simulink model "quad_sim_outerloop_multiple_UAVs_pyramid"  (R2017a)
settings: Solver=VariableStepAuto  StartTime=0.0  StopTime=250  FixedStep=0.025  MaxStep=0.03  MinStep=0.02  RelTol=1e-3  EnableMultiTasking=on
InitFcn:
  | setup_gains
  | % --- Outer loop gains --------
  | %P_X=9.44;   I_X=0.23;  D_X=2.36;
  | %P_Y=9.33;   I_Y=0.18;  D_Y=1.54;
  | % --------------------------
  | 
  | %CARLA TUNNED PID
  | %P_Z = 51.037;       I_Z = 43.051;        D_Z = 11.771;
  | %P_Z = 0.5;       I_Z = 0.15;        D_Z = 0.2;
  | %P_Z = 32.55;       I_Z = 9.82;        D_Z = 4.65 ;
  | 
  | global clientID;
  | clientID=-1;
values from neighbouring files (symbols this model uses):
  End_POS_pyramid = [ 0.3000 1.3000 0.000 ... (first row only)    [setup_gains.m]
  Kd_az = 0.001    [setup_gains.m]
  Kd_px = 0.5    [setup_gains.m]
  Kd_py = 0.5    [setup_gains.m]
  Kd_pz = 0.025    [setup_gains.m]
  Kd_vx = 2    [setup_gains.m]
  Kd_vy = 2    [setup_gains.m]
  Kd_vz = 0.05    [setup_gains.m]
  Ki_az = 0.01    [setup_gains.m]
  Ki_px = 0.001    [setup_gains.m]
  Ki_py = 0.001    [setup_gains.m]
  Ki_pz = 0.001    [setup_gains.m]
  Ki_vx = 0.1    [setup_gains.m]
  Ki_vy = 0.1    [setup_gains.m]
  Ki_vz = 2.5    [setup_gains.m]
  Kp_az = 0.75    [setup_gains.m]
  Kp_px = 1    [setup_gains.m]
  Kp_py = 1    [setup_gains.m]
  Kp_pz = 0.5    [setup_gains.m]
  Kp_vx = 15.00    (= 15)    [setup_gains.m]
  Kp_vy = 15.00    (= 15)    [setup_gains.m]
  Kp_vz = 5    [setup_gains.m]
  Start_POS = [ 0.0 0.00 1.00 ... (first row only)    [setup_gains.m]
undefined symbols (not defined in the file or in its folder): W, X, Y, Z
libraries: robotlib x27, dspindex x27, dspsigops x27, simulink x27
(part 1 of 3)
settings Model: Creator=Kleber Cabral  LastModifiedBy=Kleber Cabral
settings DataIOCC: SaveFormat=Array
settings OptimizationCC: LifeSpan=inf
settings DebuggingCC: SolverPrmCheckMsg=warning  SFUnexpectedBacktrackingDiag=warning  SFNoUnconditionalDefaultTransitionDiag=warning  SFExecutionAtInitializationDiag=none
settings HardwareCC: ProdBitPerPointer=32  ProdBitPerSizeT=32  ProdBitPerPtrDiffT=32  ProdLargestAtomicFloat=None  ProdIntDivRoundTo=Undefined  ProdEndianess=Unspecified  ProdWordSize=32  ProdHWDeviceType=32-bit Generic
settings ModelReferenceCC: PropagateSignalLabelsOutOfModel=off
settings GRTTargetCC: TargetLangStandard=C89/C90 (ANSI)  GeneratePreprocessorConditionals=Disable all
settings ConfigComp: CovMetricSettings=dw  CovHtmlReporting=on  CovSaveCumulativeToWorkspaceVar=on  CovSaveSingleToWorkspaceVar=on  CovExternalEMLEnable=off  CovSFcnEnable=off

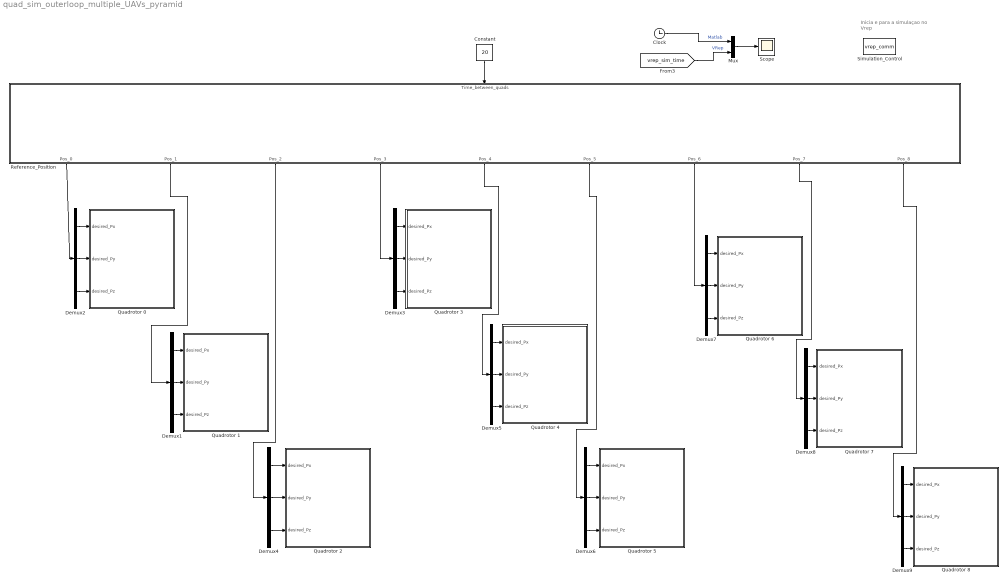
== system quad_sim_outerloop_multiple_UAVs_pyramid ==
  note: Inicia e para a simulaçao no Vrep
  Clock : Clock
  Constant : Constant  Value=20
  Demux{1..9} (9 alike) : Demux  Outputs=3
  Mux : Mux  Inputs=2
  Quadrotor 0 : Subsystem
  Quadrotor 1 : Subsystem
  Quadrotor 2 : Subsystem
  Quadrotor 3 : Subsystem
  Quadrotor 4 : Subsystem
  Quadrotor 5 : Subsystem
  Quadrotor 6 : Subsystem
  Quadrotor 7 : Subsystem
  Quadrotor 8 : Subsystem
  Reference_Position : Subsystem
  Scope : Scope
  Simulation_Control : S-Function  FunctionName=vrep_comm  SFunctionDeploymentMode=off  EnableBusSupport=off
  wires:
  Demux3/1 -> Quadrotor 3/1(desired_Px)
  Demux3/2 -> Quadrotor 3/2(desired_Py)
  Demux3/3 -> Quadrotor 3/3(desired_Pz)
  Reference_Position/4(Pos_3) -> Demux3/1
  Constant/1 -> Reference_Position/1(Time_between_quads)
  Demux1/1 -> Quadrotor 1/1(desired_Px)
  Demux1/2 -> Quadrotor 1/2(desired_Py)
  Demux1/3 -> Quadrotor 1/3(desired_Pz)
  Demux2/1 -> Quadrotor 0/1(desired_Px)
  Demux2/2 -> Quadrotor 0/2(desired_Py)
  Demux2/3 -> Quadrotor 0/3(desired_Pz)
  Reference_Position/1(Pos_0) -> Demux2/1
  Reference_Position/2(Pos_1) -> Demux1/1
  Demux4/1 -> Quadrotor 2/1(desired_Px)
  Demux4/2 -> Quadrotor 2/2(desired_Py)
  Demux4/3 -> Quadrotor 2/3(desired_Pz)
  Reference_Position/3(Pos_2) -> Demux4/1
  Demux5/1 -> Quadrotor 4/1(desired_Px)
  Demux5/2 -> Quadrotor 4/2(desired_Py)
  Demux5/3 -> Quadrotor 4/3(desired_Pz)
  Reference_Position/5(Pos_4) -> Demux5/1
  Demux6/1 -> Quadrotor 5/1(desired_Px)
  Demux6/2 -> Quadrotor 5/2(desired_Py)
  Demux6/3 -> Quadrotor 5/3(desired_Pz)
  Reference_Position/6(Pos_5) -> Demux6/1
  Demux7/3 -> Quadrotor 6/3(desired_Pz)
  Demux7/2 -> Quadrotor 6/2(desired_Py)
  Demux7/1 -> Quadrotor 6/1(desired_Px)
  Reference_Position/7(Pos_6) -> Demux7/1
  Demux8/1 -> Quadrotor 7/1(desired_Px)
  Demux8/2 -> Quadrotor 7/2(desired_Py)
  Demux8/3 -> Quadrotor 7/3(desired_Pz)
  Reference_Position/8(Pos_7) -> Demux8/1
  Demux9/1 -> Quadrotor 8/1(desired_Px)
  Demux9/2 -> Quadrotor 8/2(desired_Py)
  Demux9/3 -> Quadrotor 8/3(desired_Pz)
  Reference_Position/9(Pos_8) -> Demux9/1
  Mux/1 -> Scope/1
  Clock/1 -> Mux/1  "Matlab"
  [vrep_sim_time] -> Mux/2  "VRep"

== system quad_sim_outerloop_multiple_UAVs_pyramid/Quadrotor 0 ==
  desired_Px : Inport
  desired_Py : Inport  Port=2
  desired_Pz : Inport  Port=3
  Bus Creator1 : BusCreator  Inputs=3
  Bus Creator2 : BusCreator  Inputs=3
  Bus Selector1 : BusSelector  OutputSignals=Px,Py,Pz
  Bus Selector2 : BusSelector  OutputSignals=Vx,Vy,Vz
  Mux1 : Mux  Inputs=3
  Mux8 : Mux  Inputs=3
  Outer Control Loop : Subsystem
  Pulse Generator : DiscretePulseGenerator  PulseType=Time based  Period=0.1  PulseWidth=20
  Quadrirrotor Communication : Subsystem
  Sample and Hold : dspsigops/Sample and Hold  trig=Rising edge  initCond=0  latchinput=off
  Sample and Hold1 : dspsigops/Sample and Hold  trig=Rising edge  initCond=0  latchinput=off
  Sample and Hold2 : dspsigops/Sample and Hold  trig=Rising edge  initCond=0  latchinput=off
  TURNOFF_UAV : Subsystem
  Terminator1 : Terminator
  yaw : Constant  Value=0
  tag scope: vrep_sim_time=global
  wires:
  Quadrirrotor Communication/8(quad_acc_y) -> Terminator1/1  "Ay"
  [AccelerationZ0] -> Outer Control Loop/10(actual_Az)
  Quadrirrotor Communication/9(quad_acc_z) -> [AccelerationZ0]  "Az"
  yaw/1 -> Outer Control Loop/11(Desired_Yaw)
  Pulse Generator/1 -> Sample and Hold/Trigger, Sample and Hold1/Trigger, Sample and Hold2/Trigger
  Outer Control Loop/3(yaw_ctrl) -> Sample and Hold2/1
  Outer Control Loop/2(pitch_ctrl) -> Sample and Hold1/1
  Outer Control Loop/1(roll_ctrl) -> Sample and Hold/1
  desired_Py/1 -> Mux8/2, Outer Control Loop/2(desired_Py)
  desired_Px/1 -> Mux8/1, Outer Control Loop/1(desired_Px)
  desired_Pz/1 -> Mux8/3, Outer Control Loop/3(desired_Pz)
  [Position0] -> Bus Selector1/1
  Bus Selector1/3 -> Mux1/3, Outer Control Loop/6(actual_Pz)  "<Pz>"
  Bus Selector1/2 -> Outer Control Loop/5(actual_Py), Mux1/2  "<Py>"
  Bus Selector1/1 -> Outer Control Loop/4(actual_Px), Mux1/1  "<Px>"
  Quadrirrotor Communication/4(quad_vel_x) -> Bus Creator1/1  "Vx"
  Quadrirrotor Communication/5(quad_vel_y) -> Bus Creator1/2  "Vy"
  Quadrirrotor Communication/6(quad_vel_z) -> Bus Creator1/3  "Vz"
  Bus Creator1/1 -> [Velocity0]
  Quadrirrotor Communication/3(quad_pos_z) -> Bus Creator2/3  "Pz"
  Quadrirrotor Communication/2(quad_pos_y) -> Bus Creator2/2  "Py"
  Quadrirrotor Communication/1(quad_pos_x) -> Bus Creator2/1  "Px"
  Bus Creator2/1 -> [Position0]
  [Velocity0] -> Bus Selector2/1
  Bus Selector2/3 -> Outer Control Loop/9(actual_Vz)  "<Vz>"
  Bus Selector2/2 -> Outer Control Loop/8(actual_Vy)  "<Vy>"
  Bus Selector2/1 -> Outer Control Loop/7(actual_Vx)  "<Vx>"
  Sample and Hold/1 -> TURNOFF_UAV/3(roll_in)
  Sample and Hold1/1 -> TURNOFF_UAV/4(pitch_in)
  Sample and Hold2/1 -> TURNOFF_UAV/5(yaw_in)
  Outer Control Loop/4(altura_ctrl) -> TURNOFF_UAV/6(height_in)
  TURNOFF_UAV/1(roll_out) -> Quadrirrotor Communication/1(roll)
  TURNOFF_UAV/2(pitch_out) -> Quadrirrotor Communication/2(pitch)
  TURNOFF_UAV/3(yaw_out) -> Quadrirrotor Communication/3(yaw)
  TURNOFF_UAV/4(height_out) -> Quadrirrotor Communication/4(throttle)
  Mux8/1 -> TURNOFF_UAV/1(desired)
  Mux1/1 -> TURNOFF_UAV/2(actual)
  Quadrirrotor Communication/7(quad_acc_x) -> [vrep_sim_time]  "Ax"

== system quad_sim_outerloop_multiple_UAVs_pyramid/Quadrotor 1 ==
  desired_Px : Inport
  desired_Py : Inport  Port=2
  desired_Pz : Inport  Port=3
  Bus Creator1 : BusCreator  Inputs=3
  Bus Creator2 : BusCreator  Inputs=3
  Bus Selector1 : BusSelector  OutputSignals=Px,Py,Pz
  Bus Selector2 : BusSelector  OutputSignals=Vx,Vy,Vz
  Mux1 : Mux  Inputs=3
  Mux8 : Mux  Inputs=3
  Outer Control Loop : Subsystem
  Pulse Generator : DiscretePulseGenerator  PulseType=Time based  Period=0.1  PulseWidth=20
  Quadrirrotor Communication : Subsystem
  Sample and Hold : dspsigops/Sample and Hold  trig=Rising edge  initCond=0  latchinput=off
  Sample and Hold1 : dspsigops/Sample and Hold  trig=Rising edge  initCond=0  latchinput=off
  Sample and Hold2 : dspsigops/Sample and Hold  trig=Rising edge  initCond=0  latchinput=off
  TURNOFF_UAV : Subsystem
  Terminator : Terminator
  Terminator1 : Terminator
  yaw : Constant  Value=0
  wires:
  Bus Selector2/1 -> Outer Control Loop/7(actual_Vx)  "<Vx>"
  Bus Selector2/2 -> Outer Control Loop/8(actual_Vy)  "<Vy>"
  Bus Selector2/3 -> Outer Control Loop/9(actual_Vz)  "<Vz>"
  [Velocity1] -> Bus Selector2/1
  Bus Creator2/1 -> [Position1]
  Quadrirrotor Communication/1(quad_pos_x) -> Bus Creator2/1  "Px"
  Quadrirrotor Communication/2(quad_pos_y) -> Bus Creator2/2  "Py"
  Quadrirrotor Communication/3(quad_pos_z) -> Bus Creator2/3  "Pz"
  Bus Creator1/1 -> [Velocity1]
  Quadrirrotor Communication/6(quad_vel_z) -> Bus Creator1/3  "Vz"
  Quadrirrotor Communication/5(quad_vel_y) -> Bus Creator1/2  "Vy"
  Quadrirrotor Communication/4(quad_vel_x) -> Bus Creator1/1  "Vx"
  [Position1] -> Bus Selector1/1
  Outer Control Loop/4(altura_ctrl) -> TURNOFF_UAV/6(height_in)
  desired_Px/1 -> Mux8/1, Outer Control Loop/1(desired_Px)
  Outer Control Loop/1(roll_ctrl) -> Sample and Hold/1
  Outer Control Loop/2(pitch_ctrl) -> Sample and Hold1/1
  Outer Control Loop/3(yaw_ctrl) -> Sample and Hold2/1
  Pulse Generator/1 -> Sample and Hold2/Trigger, Sample and Hold1/Trigger, Sample and Hold/Trigger
  yaw/1 -> Outer Control Loop/11(Desired_Yaw)
  Quadrirrotor Communication/9(quad_acc_z) -> [AccelerationZ1]  "Az"
  [AccelerationZ1] -> Outer Control Loop/10(actual_Az)
  Quadrirrotor Communication/8(quad_acc_y) -> Terminator1/1  "Ay"
  Quadrirrotor Communication/7(quad_acc_x) -> Terminator/1  "Ax"
  Mux1/1 -> TURNOFF_UAV/2(actual)
  Bus Selector1/1 -> Mux1/1, Outer Control Loop/4(actual_Px)  "<Px>"
  desired_Pz/1 -> Mux8/3, Outer Control Loop/3(desired_Pz)
  desired_Py/1 -> Mux8/2, Outer Control Loop/2(desired_Py)
  Mux8/1 -> TURNOFF_UAV/1(desired)
  Bus Selector1/2 -> Mux1/2, Outer Control Loop/5(actual_Py)  "<Py>"
  Bus Selector1/3 -> Mux1/3, Outer Control Loop/6(actual_Pz)  "<Pz>"
  Sample and Hold2/1 -> TURNOFF_UAV/5(yaw_in)
  Sample and Hold1/1 -> TURNOFF_UAV/4(pitch_in)
  Sample and Hold/1 -> TURNOFF_UAV/3(roll_in)
  TURNOFF_UAV/1(roll_out) -> Quadrirrotor Communication/1(roll)
  TURNOFF_UAV/2(pitch_out) -> Quadrirrotor Communication/2(pitch)
  TURNOFF_UAV/3(yaw_out) -> Quadrirrotor Communication/3(yaw)
  TURNOFF_UAV/4(height_out) -> Quadrirrotor Communication/4(throttle)

== system quad_sim_outerloop_multiple_UAVs_pyramid/Quadrotor 2 ==
  desired_Px : Inport
  desired_Py : Inport  Port=2
  desired_Pz : Inport  Port=3
  Bus Creator1 : BusCreator  Inputs=3
  Bus Creator2 : BusCreator  Inputs=3
  Bus Selector1 : BusSelector  OutputSignals=Px,Py,Pz
  Bus Selector2 : BusSelector  OutputSignals=Vx,Vy,Vz
  Mux1 : Mux  Inputs=3
  Mux8 : Mux  Inputs=3
  Outer Control Loop : Subsystem
  Pulse Generator : DiscretePulseGenerator  PulseType=Time based  Period=0.1  PulseWidth=20
  Quadrirrotor Communication : Subsystem
  Sample and Hold : dspsigops/Sample and Hold  trig=Rising edge  initCond=0  latchinput=off
  Sample and Hold1 : dspsigops/Sample and Hold  trig=Rising edge  initCond=0  latchinput=off
  Sample and Hold2 : dspsigops/Sample and Hold  trig=Rising edge  initCond=0  latchinput=off
  TURNOFF_UAV : Subsystem
  Terminator : Terminator
  Terminator1 : Terminator
  yaw : Constant  Value=0
  wires:
  Quadrirrotor Communication/7(quad_acc_x) -> Terminator/1  "Ax"
  Quadrirrotor Communication/8(quad_acc_y) -> Terminator1/1  "Ay"
  [AccelerationZ2] -> Outer Control Loop/10(actual_Az)
  Quadrirrotor Communication/9(quad_acc_z) -> [AccelerationZ2]  "Az"
  yaw/1 -> Outer Control Loop/11(Desired_Yaw)
  Pulse Generator/1 -> Sample and Hold/Trigger, Sample and Hold1/Trigger, Sample and Hold2/Trigger
  Outer Control Loop/3(yaw_ctrl) -> Sample and Hold2/1
  Outer Control Loop/2(pitch_ctrl) -> Sample and Hold1/1
  Outer Control Loop/1(roll_ctrl) -> Sample and Hold/1
  desired_Px/1 -> Mux8/1, Outer Control Loop/1(desired_Px)
  [Position2] -> Bus Selector1/1
  Quadrirrotor Communication/4(quad_vel_x) -> Bus Creator1/1  "Vx"
  Quadrirrotor Communication/5(quad_vel_y) -> Bus Creator1/2  "Vy"
  Quadrirrotor Communication/6(quad_vel_z) -> Bus Creator1/3  "Vz"
  Bus Creator1/1 -> [Velocity2]
  Quadrirrotor Communication/3(quad_pos_z) -> Bus Creator2/3  "Pz"
  Quadrirrotor Communication/2(quad_pos_y) -> Bus Creator2/2  "Py"
  Quadrirrotor Communication/1(quad_pos_x) -> Bus Creator2/1  "Px"
  Bus Creator2/1 -> [Position2]
  [Velocity2] -> Bus Selector2/1
  Bus Selector2/3 -> Outer Control Loop/9(actual_Vz)  "<Vz>"
  Bus Selector2/2 -> Outer Control Loop/8(actual_Vy)  "<Vy>"
  Bus Selector2/1 -> Outer Control Loop/7(actual_Vx)  "<Vx>"
  Bus Selector1/1 -> Mux1/1, Outer Control Loop/4(actual_Px)  "<Px>"
  desired_Pz/1 -> Mux8/3, Outer Control Loop/3(desired_Pz)
  desired_Py/1 -> Mux8/2, Outer Control Loop/2(desired_Py)
  Bus Selector1/2 -> Mux1/2, Outer Control Loop/5(actual_Py)  "<Py>"
  Mux1/1 -> TURNOFF_UAV/2(actual)
  Mux8/1 -> TURNOFF_UAV/1(desired)
  Bus Selector1/3 -> Mux1/3, Outer Control Loop/6(actual_Pz)  "<Pz>"
  Sample and Hold/1 -> TURNOFF_UAV/3(roll_in)
  Sample and Hold1/1 -> TURNOFF_UAV/4(pitch_in)
  Sample and Hold2/1 -> TURNOFF_UAV/5(yaw_in)
  Outer Control Loop/4(altura_ctrl) -> TURNOFF_UAV/6(height_in)
  TURNOFF_UAV/4(height_out) -> Quadrirrotor Communication/4(throttle)
  TURNOFF_UAV/3(yaw_out) -> Quadrirrotor Communication/3(yaw)
  TURNOFF_UAV/2(pitch_out) -> Quadrirrotor Communication/2(pitch)
  TURNOFF_UAV/1(roll_out) -> Quadrirrotor Communication/1(roll)

== system quad_sim_outerloop_multiple_UAVs_pyramid/Quadrotor 3 ==
  desired_Px : Inport
  desired_Py : Inport  Port=2
  desired_Pz : Inport  Port=3
  Bus Creator1 : BusCreator  Inputs=3
  Bus Creator2 : BusCreator  Inputs=3
  Bus Selector1 : BusSelector  OutputSignals=Px,Py,Pz
  Bus Selector2 : BusSelector  OutputSignals=Vx,Vy,Vz
  Mux1 : Mux  Inputs=3
  Mux8 : Mux  Inputs=3
  Outer Control Loop : Subsystem
  Pulse Generator : DiscretePulseGenerator  PulseType=Time based  Period=0.1  PulseWidth=20
  Quadrirrotor Communication : Subsystem
  Sample and Hold : dspsigops/Sample and Hold  trig=Rising edge  initCond=0  latchinput=off
  Sample and Hold1 : dspsigops/Sample and Hold  trig=Rising edge  initCond=0  latchinput=off
  Sample and Hold2 : dspsigops/Sample and Hold  trig=Rising edge  initCond=0  latchinput=off
  Subsystem1 : Subsystem
  Terminator : Terminator
  Terminator1 : Terminator
  yaw : Constant  Value=0
  wires:
  Bus Selector2/1 -> Outer Control Loop/7(actual_Vx)  "<Vx>"
  Bus Selector2/2 -> Outer Control Loop/8(actual_Vy)  "<Vy>"
  Bus Selector2/3 -> Outer Control Loop/9(actual_Vz)  "<Vz>"
  [Velocity3] -> Bus Selector2/1
  Bus Creator2/1 -> [Position3]
  Quadrirrotor Communication/1(quad_pos_x) -> Bus Creator2/1  "Px"
  Quadrirrotor Communication/2(quad_pos_y) -> Bus Creator2/2  "Py"
  Quadrirrotor Communication/3(quad_pos_z) -> Bus Creator2/3  "Pz"
  Bus Creator1/1 -> [Velocity3]
  Quadrirrotor Communication/6(quad_vel_z) -> Bus Creator1/3  "Vz"
  Quadrirrotor Communication/5(quad_vel_y) -> Bus Creator1/2  "Vy"
  Quadrirrotor Communication/4(quad_vel_x) -> Bus Creator1/1  "Vx"
  [Position3] -> Bus Selector1/1
  desired_Px/1 -> Mux8/1, Outer Control Loop/1(desired_Px)
  Outer Control Loop/1(roll_ctrl) -> Sample and Hold/1
  Outer Control Loop/2(pitch_ctrl) -> Sample and Hold1/1
  Outer Control Loop/3(yaw_ctrl) -> Sample and Hold2/1
  Pulse Generator/1 -> Sample and Hold2/Trigger, Sample and Hold1/Trigger, Sample and Hold/Trigger
  yaw/1 -> Outer Control Loop/11(Desired_Yaw)
  Quadrirrotor Communication/9(quad_acc_z) -> [AccelerationZ3]  "Az"
  [AccelerationZ3] -> Outer Control Loop/10(actual_Az)
  Quadrirrotor Communication/8(quad_acc_y) -> Terminator1/1  "Ay"
  Quadrirrotor Communication/7(quad_acc_x) -> Terminator/1  "Ax"
  Bus Selector1/1 -> Mux1/1, Outer Control Loop/4(actual_Px)  "<Px>"
  desired_Pz/1 -> Mux8/3, Outer Control Loop/3(desired_Pz)
  desired_Py/1 -> Mux8/2, Outer Control Loop/2(desired_Py)
  Bus Selector1/2 -> Mux1/2, Outer Control Loop/5(actual_Py)  "<Py>"
  Mux1/1 -> Subsystem1/2(actual)
  Mux8/1 -> Subsystem1/1(desired)
  Bus Selector1/3 -> Mux1/3, Outer Control Loop/6(actual_Pz)  "<Pz>"
  Sample and Hold2/1 -> Subsystem1/5(yaw_in)
  Sample and Hold1/1 -> Subsystem1/4(pitch_in)
  Sample and Hold/1 -> Subsystem1/3(roll_in)
  Outer Control Loop/4(altura_ctrl) -> Subsystem1/6(height_in)
  Subsystem1/4(height_out) -> Quadrirrotor Communication/4(throttle)
  Subsystem1/3(yaw_out) -> Quadrirrotor Communication/3(yaw)
  Subsystem1/2(pitch_out) -> Quadrirrotor Communication/2(pitch)
  Subsystem1/1(roll_out) -> Quadrirrotor Communication/1(roll)

== system quad_sim_outerloop_multiple_UAVs_pyramid/Quadrotor 4 ==
  desired_Px : Inport
  desired_Py : Inport  Port=2
  desired_Pz : Inport  Port=3
  Bus Creator1 : BusCreator  Inputs=3
  Bus Creator2 : BusCreator  Inputs=3
  Bus Selector1 : BusSelector  OutputSignals=Px,Py,Pz
  Bus Selector2 : BusSelector  OutputSignals=Vx,Vy,Vz
  Mux1 : Mux  Inputs=3
  Mux8 : Mux  Inputs=3
  Outer Control Loop : Subsystem
  Pulse Generator : DiscretePulseGenerator  PulseType=Time based  Period=0.1  PulseWidth=20
  Quadrirrotor Communication : Subsystem
  Sample and Hold : dspsigops/Sample and Hold  trig=Rising edge  initCond=0  latchinput=off
  Sample and Hold1 : dspsigops/Sample and Hold  trig=Rising edge  initCond=0  latchinput=off
  Sample and Hold2 : dspsigops/Sample and Hold  trig=Rising edge  initCond=0  latchinput=off
  Subsystem1 : Subsystem
  Terminator : Terminator
  Terminator1 : Terminator
  yaw : Constant  Value=0
  wires:
  Bus Selector2/1 -> Outer Control Loop/7(actual_Vx)  "<Vx>"
  Bus Selector2/2 -> Outer Control Loop/8(actual_Vy)  "<Vy>"
  Bus Selector2/3 -> Outer Control Loop/9(actual_Vz)  "<Vz>"
  [Velocity4] -> Bus Selector2/1
  Bus Creator2/1 -> [Position4]
  Quadrirrotor Communication/1(quad_pos_x) -> Bus Creator2/1  "Px"
  Quadrirrotor Communication/2(quad_pos_y) -> Bus Creator2/2  "Py"
  Quadrirrotor Communication/3(quad_pos_z) -> Bus Creator2/3  "Pz"
  Bus Creator1/1 -> [Velocity4]
  Quadrirrotor Communication/6(quad_vel_z) -> Bus Creator1/3  "Vz"
  Quadrirrotor Communication/5(quad_vel_y) -> Bus Creator1/2  "Vy"
  Quadrirrotor Communication/4(quad_vel_x) -> Bus Creator1/1  "Vx"
  [Position4] -> Bus Selector1/1
  desired_Px/1 -> Mux8/1, Outer Control Loop/1(desired_Px)
  Outer Control Loop/1(roll_ctrl) -> Sample and Hold/1
  Outer Control Loop/2(pitch_ctrl) -> Sample and Hold1/1
  Outer Control Loop/3(yaw_ctrl) -> Sample and Hold2/1
  Pulse Generator/1 -> Sample and Hold2/Trigger, Sample and Hold1/Trigger, Sample and Hold/Trigger
  yaw/1 -> Outer Control Loop/11(Desired_Yaw)
  Quadrirrotor Communication/9(quad_acc_z) -> [AccelerationZ4]  "Az"
  [AccelerationZ4] -> Outer Control Loop/10(actual_Az)
  Quadrirrotor Communication/8(quad_acc_y) -> Terminator1/1  "Ay"
  Quadrirrotor Communication/7(quad_acc_x) -> Terminator/1  "Ax"
  Bus Selector1/1 -> Mux1/1, Outer Control Loop/4(actual_Px)  "<Px>"
  desired_Pz/1 -> Mux8/3, Outer Control Loop/3(desired_Pz)
  desired_Py/1 -> Mux8/2, Outer Control Loop/2(desired_Py)
  Bus Selector1/2 -> Mux1/2, Outer Control Loop/5(actual_Py)  "<Py>"
  Mux1/1 -> Subsystem1/2(actual)
  Mux8/1 -> Subsystem1/1(desired)
  Bus Selector1/3 -> Mux1/3, Outer Control Loop/6(actual_Pz)  "<Pz>"
  Sample and Hold2/1 -> Subsystem1/5(yaw_in)
  Sample and Hold1/1 -> Subsystem1/4(pitch_in)
  Sample and Hold/1 -> Subsystem1/3(roll_in)
  Outer Control Loop/4(altura_ctrl) -> Subsystem1/6(height_in)
  Subsystem1/4(height_out) -> Quadrirrotor Communication/4(throttle)
  Subsystem1/3(yaw_out) -> Quadrirrotor Communication/3(yaw)
  Subsystem1/2(pitch_out) -> Quadrirrotor Communication/2(pitch)
  Subsystem1/1(roll_out) -> Quadrirrotor Communication/1(roll)

== system quad_sim_outerloop_multiple_UAVs_pyramid/Quadrotor 5 ==
  desired_Px : Inport
  desired_Py : Inport  Port=2
  desired_Pz : Inport  Port=3
  Bus Creator1 : BusCreator  Inputs=3
  Bus Creator2 : BusCreator  Inputs=3
  Bus Selector1 : BusSelector  OutputSignals=Px,Py,Pz
  Bus Selector2 : BusSelector  OutputSignals=Vx,Vy,Vz
  Mux1 : Mux  Inputs=3
  Mux8 : Mux  Inputs=3
  Outer Control Loop : Subsystem
  Pulse Generator : DiscretePulseGenerator  PulseType=Time based  Period=0.1  PulseWidth=20
  Quadrirrotor Communication : Subsystem
  Sample and Hold : dspsigops/Sample and Hold  trig=Rising edge  initCond=0  latchinput=off
  Sample and Hold1 : dspsigops/Sample and Hold  trig=Rising edge  initCond=0  latchinput=off
  Sample and Hold2 : dspsigops/Sample and Hold  trig=Rising edge  initCond=0  latchinput=off
  Subsystem1 : Subsystem
  Terminator : Terminator
  Terminator1 : Terminator
  yaw : Constant  Value=0
  wires:
  Quadrirrotor Communication/7(quad_acc_x) -> Terminator/1  "Ax"
  Quadrirrotor Communication/8(quad_acc_y) -> Terminator1/1  "Ay"
  [AccelerationZ5] -> Outer Control Loop/10(actual_Az)
  Quadrirrotor Communication/9(quad_acc_z) -> [AccelerationZ5]  "Az"
  yaw/1 -> Outer Control Loop/11(Desired_Yaw)
  Pulse Generator/1 -> Sample and Hold/Trigger, Sample and Hold1/Trigger, Sample and Hold2/Trigger
  Outer Control Loop/3(yaw_ctrl) -> Sample and Hold2/1
  Outer Control Loop/2(pitch_ctrl) -> Sample and Hold1/1
  Outer Control Loop/1(roll_ctrl) -> Sample and Hold/1
  [Position5] -> Bus Selector1/1
  Quadrirrotor Communication/4(quad_vel_x) -> Bus Creator1/1  "Vx"
  Quadrirrotor Communication/5(quad_vel_y) -> Bus Creator1/2  "Vy"
  Quadrirrotor Communication/6(quad_vel_z) -> Bus Creator1/3  "Vz"
  Bus Creator1/1 -> [Velocity5]
  Quadrirrotor Communication/3(quad_pos_z) -> Bus Creator2/3  "Pz"
  Quadrirrotor Communication/2(quad_pos_y) -> Bus Creator2/2  "Py"
  Quadrirrotor Communication/1(quad_pos_x) -> Bus Creator2/1  "Px"
  Bus Creator2/1 -> [Position5]
  [Velocity5] -> Bus Selector2/1
  Bus Selector2/3 -> Outer Control Loop/9(actual_Vz)  "<Vz>"
  Bus Selector2/2 -> Outer Control Loop/8(actual_Vy)  "<Vy>"
  Bus Selector2/1 -> Outer Control Loop/7(actual_Vx)  "<Vx>"
  Bus Selector1/1 -> Mux1/1, Outer Control Loop/4(actual_Px)  "<Px>"
  desired_Pz/1 -> Mux8/3, Outer Control Loop/3(desired_Pz)
  desired_Py/1 -> Mux8/2, Outer Control Loop/2(desired_Py)
  Bus Selector1/2 -> Mux1/2, Outer Control Loop/5(actual_Py)  "<Py>"
  Mux1/1 -> Subsystem1/2(actual)
  Mux8/1 -> Subsystem1/1(desired)
  Bus Selector1/3 -> Mux1/3, Outer Control Loop/6(actual_Pz)  "<Pz>"
  Sample and Hold2/1 -> Subsystem1/5(yaw_in)
  Sample and Hold1/1 -> Subsystem1/4(pitch_in)
  Sample and Hold/1 -> Subsystem1/3(roll_in)
  Outer Control Loop/4(altura_ctrl) -> Subsystem1/6(height_in)
  Subsystem1/4(height_out) -> Quadrirrotor Communication/4(throttle)
  Subsystem1/3(yaw_out) -> Quadrirrotor Communication/3(yaw)
  Subsystem1/2(pitch_out) -> Quadrirrotor Communication/2(pitch)
  Subsystem1/1(roll_out) -> Quadrirrotor Communication/1(roll)
  desired_Px/1 -> Mux8/1, Outer Control Loop/1(desired_Px)

== system quad_sim_outerloop_multiple_UAVs_pyramid/Quadrotor 6 ==
  desired_Px : Inport
  desired_Py : Inport  Port=2
  desired_Pz : Inport  Port=3
  Bus Creator1 : BusCreator  Inputs=3
  Bus Creator2 : BusCreator  Inputs=3
  Bus Selector1 : BusSelector  OutputSignals=Px,Py,Pz
  Bus Selector2 : BusSelector  OutputSignals=Vx,Vy,Vz
  Mux1 : Mux  Inputs=3
  Mux8 : Mux  Inputs=3
  Outer Control Loop : Subsystem
  Pulse Generator : DiscretePulseGenerator  PulseType=Time based  Period=0.1  PulseWidth=20
  Quadrirrotor Communication : Subsystem
  Sample and Hold : dspsigops/Sample and Hold  trig=Rising edge  initCond=0  latchinput=off
  Sample and Hold1 : dspsigops/Sample and Hold  trig=Rising edge  initCond=0  latchinput=off
  Sample and Hold2 : dspsigops/Sample and Hold  trig=Rising edge  initCond=0  latchinput=off
  Subsystem1 : Subsystem
  Terminator : Terminator
  Terminator1 : Terminator
  yaw : Constant  Value=0
  wires:
  Bus Selector2/1 -> Outer Control Loop/7(actual_Vx)  "<Vx>"
  Bus Selector2/2 -> Outer Control Loop/8(actual_Vy)  "<Vy>"
  Bus Selector2/3 -> Outer Control Loop/9(actual_Vz)  "<Vz>"
  [Velocity6] -> Bus Selector2/1
  Bus Creator2/1 -> [Position6]
  Quadrirrotor Communication/1(quad_pos_x) -> Bus Creator2/1  "Px"
  Quadrirrotor Communication/2(quad_pos_y) -> Bus Creator2/2  "Py"
  Quadrirrotor Communication/3(quad_pos_z) -> Bus Creator2/3  "Pz"
  Bus Creator1/1 -> [Velocity6]
  Quadrirrotor Communication/6(quad_vel_z) -> Bus Creator1/3  "Vz"
  Quadrirrotor Communication/5(quad_vel_y) -> Bus Creator1/2  "Vy"
  Quadrirrotor Communication/4(quad_vel_x) -> Bus Creator1/1  "Vx"
  [Position6] -> Bus Selector1/1
  desired_Pz/1 -> Outer Control Loop/3(desired_Pz), Mux8/3
  desired_Py/1 -> Mux8/2, Outer Control Loop/2(desired_Py)
  Outer Control Loop/1(roll_ctrl) -> Sample and Hold/1
  Outer Control Loop/2(pitch_ctrl) -> Sample and Hold1/1
  Outer Control Loop/3(yaw_ctrl) -> Sample and Hold2/1
  Pulse Generator/1 -> Sample and Hold2/Trigger, Sample and Hold1/Trigger, Sample and Hold/Trigger
  yaw/1 -> Outer Control Loop/11(Desired_Yaw)
  Quadrirrotor Communication/9(quad_acc_z) -> [AccelerationZ6]  "Az"
  [AccelerationZ6] -> Outer Control Loop/10(actual_Az)
  Quadrirrotor Communication/8(quad_acc_y) -> Terminator1/1  "Ay"
  Quadrirrotor Communication/7(quad_acc_x) -> Terminator/1  "Ax"
  Bus Selector1/1 -> Mux1/1, Outer Control Loop/4(actual_Px)  "<Px>"
  Bus Selector1/2 -> Mux1/2, Outer Control Loop/5(actual_Py)  "<Py>"
  Mux1/1 -> Subsystem1/2(actual)
  Mux8/1 -> Subsystem1/1(desired)
  Bus Selector1/3 -> Mux1/3, Outer Control Loop/6(actual_Pz)  "<Pz>"
  desired_Px/1 -> Mux8/1, Outer Control Loop/1(desired_Px)
  Sample and Hold2/1 -> Subsystem1/5(yaw_in)
  Sample and Hold1/1 -> Subsystem1/4(pitch_in)
  Sample and Hold/1 -> Subsystem1/3(roll_in)
  Outer Control Loop/4(altura_ctrl) -> Subsystem1/6(height_in)
  Subsystem1/4(height_out) -> Quadrirrotor Communication/4(throttle)
  Subsystem1/3(yaw_out) -> Quadrirrotor Communication/3(yaw)
  Subsystem1/2(pitch_out) -> Quadrirrotor Communication/2(pitch)
  Subsystem1/1(roll_out) -> Quadrirrotor Communication/1(roll)

== system quad_sim_outerloop_multiple_UAVs_pyramid/Quadrotor 7 ==
  desired_Px : Inport
  desired_Py : Inport  Port=2
  desired_Pz : Inport  Port=3
  Bus Creator1 : BusCreator  Inputs=3
  Bus Creator2 : BusCreator  Inputs=3
  Bus Selector1 : BusSelector  OutputSignals=Px,Py,Pz
  Bus Selector2 : BusSelector  OutputSignals=Vx,Vy,Vz
  Mux1 : Mux  Inputs=3
  Mux8 : Mux  Inputs=3
  Outer Control Loop : Subsystem
  Pulse Generator : DiscretePulseGenerator  PulseType=Time based  Period=0.1  PulseWidth=20
  Quadrirrotor Communication : Subsystem
  Sample and Hold : dspsigops/Sample and Hold  trig=Rising edge  initCond=0  latchinput=off
  Sample and Hold1 : dspsigops/Sample and Hold  trig=Rising edge  initCond=0  latchinput=off
  Sample and Hold2 : dspsigops/Sample and Hold  trig=Rising edge  initCond=0  latchinput=off
  Subsystem1 : Subsystem
  Terminator : Terminator
  Terminator1 : Terminator
  yaw : Constant  Value=0
  wires:
  Quadrirrotor Communication/7(quad_acc_x) -> Terminator/1  "Ax"
  Quadrirrotor Communication/8(quad_acc_y) -> Terminator1/1  "Ay"
  [AccelerationZ7] -> Outer Control Loop/10(actual_Az)
  Quadrirrotor Communication/9(quad_acc_z) -> [AccelerationZ7]  "Az"
  yaw/1 -> Outer Control Loop/11(Desired_Yaw)
  Pulse Generator/1 -> Sample and Hold/Trigger, Sample and Hold1/Trigger, Sample and Hold2/Trigger
  Outer Control Loop/3(yaw_ctrl) -> Sample and Hold2/1
  Outer Control Loop/2(pitch_ctrl) -> Sample and Hold1/1
  Outer Control Loop/1(roll_ctrl) -> Sample and Hold/1
  desired_Py/1 -> Mux8/2, Outer Control Loop/2(desired_Py)
  desired_Px/1 -> Mux8/1, Outer Control Loop/1(desired_Px)
  desired_Pz/1 -> Mux8/3, Outer Control Loop/3(desired_Pz)
  [Position7] -> Bus Selector1/1
  Quadrirrotor Communication/4(quad_vel_x) -> Bus Creator1/1  "Vx"
  Quadrirrotor Communication/5(quad_vel_y) -> Bus Creator1/2  "Vy"
  Quadrirrotor Communication/6(quad_vel_z) -> Bus Creator1/3  "Vz"
  Bus Creator1/1 -> [Velocity7]
  Quadrirrotor Communication/3(quad_pos_z) -> Bus Creator2/3  "Pz"
  Quadrirrotor Communication/2(quad_pos_y) -> Bus Creator2/2  "Py"
  Quadrirrotor Communication/1(quad_pos_x) -> Bus Creator2/1  "Px"
  Bus Creator2/1 -> [Position7]
  [Velocity7] -> Bus Selector2/1
  Bus Selector2/3 -> Outer Control Loop/9(actual_Vz)  "<Vz>"
  Bus Selector2/2 -> Outer Control Loop/8(actual_Vy)  "<Vy>"
  Bus Selector2/1 -> Outer Control Loop/7(actual_Vx)  "<Vx>"
  Bus Selector1/1 -> Mux1/1, Outer Control Loop/4(actual_Px)  "<Px>"
  Bus Selector1/2 -> Mux1/2, Outer Control Loop/5(actual_Py)  "<Py>"
  Mux1/1 -> Subsystem1/2(actual)
  Mux8/1 -> Subsystem1/1(desired)
  Bus Selector1/3 -> Mux1/3, Outer Control Loop/6(actual_Pz)  "<Pz>"
  Sample and Hold2/1 -> Subsystem1/5(yaw_in)
  Sample and Hold1/1 -> Subsystem1/4(pitch_in)
  Sample and Hold/1 -> Subsystem1/3(roll_in)
  Outer Control Loop/4(altura_ctrl) -> Subsystem1/6(height_in)
  Subsystem1/4(height_out) -> Quadrirrotor Communication/4(throttle)
  Subsystem1/3(yaw_out) -> Quadrirrotor Communication/3(yaw)
  Subsystem1/2(pitch_out) -> Quadrirrotor Communication/2(pitch)
  Subsystem1/1(roll_out) -> Quadrirrotor Communication/1(roll)

== system quad_sim_outerloop_multiple_UAVs_pyramid/Quadrotor 8 ==
  desired_Px : Inport
  desired_Py : Inport  Port=2
  desired_Pz : Inport  Port=3
  Bus Creator1 : BusCreator  Inputs=3
  Bus Creator2 : BusCreator  Inputs=3
  Bus Selector1 : BusSelector  OutputSignals=Px,Py,Pz
  Bus Selector2 : BusSelector  OutputSignals=Vx,Vy,Vz
  Mux1 : Mux  Inputs=3
  Mux8 : Mux  Inputs=3
  Outer Control Loop : Subsystem
  Pulse Generator : DiscretePulseGenerator  PulseType=Time based  Period=0.1  PulseWidth=20
  Quadrirrotor Communication : Subsystem
  Sample and Hold : dspsigops/Sample and Hold  trig=Rising edge  initCond=0  latchinput=off
  Sample and Hold1 : dspsigops/Sample and Hold  trig=Rising edge  initCond=0  latchinput=off
  Sample and Hold2 : dspsigops/Sample and Hold  trig=Rising edge  initCond=0  latchinput=off
  Subsystem1 : Subsystem
  Terminator : Terminator
  Terminator1 : Terminator
  yaw : Constant  Value=0
  wires:
  Bus Selector2/1 -> Outer Control Loop/7(actual_Vx)  "<Vx>"
  Bus Selector2/2 -> Outer Control Loop/8(actual_Vy)  "<Vy>"
  Bus Selector2/3 -> Outer Control Loop/9(actual_Vz)  "<Vz>"
  [Velocity8] -> Bus Selector2/1
  Bus Creator2/1 -> [Position8]
  Quadrirrotor Communication/1(quad_pos_x) -> Bus Creator2/1  "Px"
  Quadrirrotor Communication/2(quad_pos_y) -> Bus Creator2/2  "Py"
  Quadrirrotor Communication/3(quad_pos_z) -> Bus Creator2/3  "Pz"
  Bus Creator1/1 -> [Velocity8]
  Quadrirrotor Communication/6(quad_vel_z) -> Bus Creator1/3  "Vz"
  Quadrirrotor Communication/5(quad_vel_y) -> Bus Creator1/2  "Vy"
  Quadrirrotor Communication/4(quad_vel_x) -> Bus Creator1/1  "Vx"
  [Position8] -> Bus Selector1/1
  desired_Pz/1 -> Mux8/3, Outer Control Loop/3(desired_Pz)
  desired_Px/1 -> Mux8/1, Outer Control Loop/1(desired_Px)
  desired_Py/1 -> Mux8/2, Outer Control Loop/2(desired_Py)
  Outer Control Loop/1(roll_ctrl) -> Sample and Hold/1
  Outer Control Loop/2(pitch_ctrl) -> Sample and Hold1/1
  Outer Control Loop/3(yaw_ctrl) -> Sample and Hold2/1
  Pulse Generator/1 -> Sample and Hold2/Trigger, Sample and Hold1/Trigger, Sample and Hold/Trigger
  yaw/1 -> Outer Control Loop/11(Desired_Yaw)
  Quadrirrotor Communication/9(quad_acc_z) -> [AccelerationZ8]  "Az"
  [AccelerationZ8] -> Outer Control Loop/10(actual_Az)
  Quadrirrotor Communication/8(quad_acc_y) -> Terminator1/1  "Ay"
  Quadrirrotor Communication/7(quad_acc_x) -> Terminator/1  "Ax"
  Bus Selector1/1 -> Mux1/1, Outer Control Loop/4(actual_Px)  "<Px>"
  Bus Selector1/2 -> Mux1/2, Outer Control Loop/5(actual_Py)  "<Py>"
  Mux1/1 -> Subsystem1/2(actual)
  Mux8/1 -> Subsystem1/1(desired)
  Bus Selector1/3 -> Mux1/3, Outer Control Loop/6(actual_Pz)  "<Pz>"
  Sample and Hold2/1 -> Subsystem1/5(yaw_in)
  Sample and Hold1/1 -> Subsystem1/4(pitch_in)
  Sample and Hold/1 -> Subsystem1/3(roll_in)
  Outer Control Loop/4(altura_ctrl) -> Subsystem1/6(height_in)
  Subsystem1/4(height_out) -> Quadrirrotor Communication/4(throttle)
  Subsystem1/3(yaw_out) -> Quadrirrotor Communication/3(yaw)
  Subsystem1/2(pitch_out) -> Quadrirrotor Communication/2(pitch)
  Subsystem1/1(roll_out) -> Quadrirrotor Communication/1(roll)

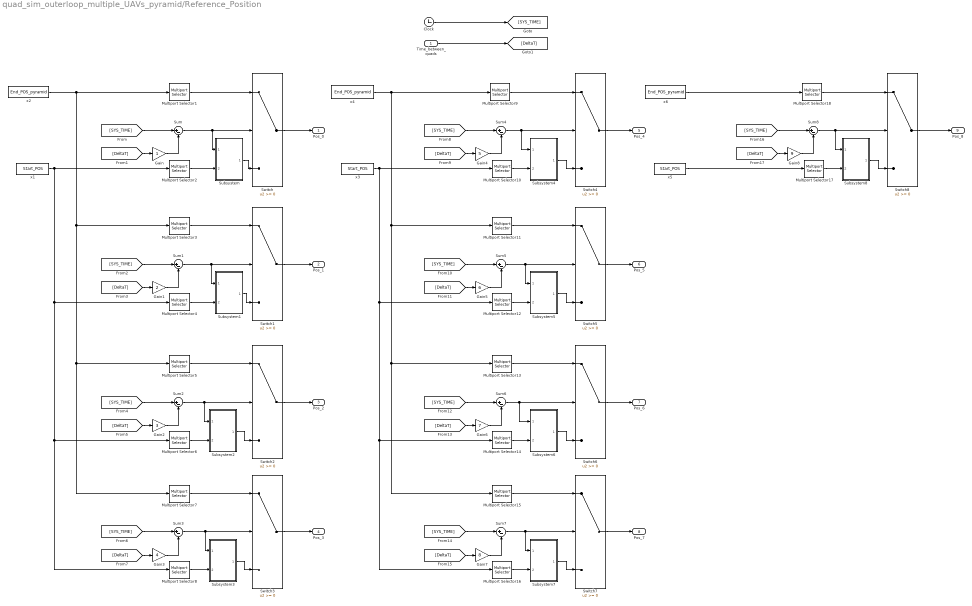
== system quad_sim_outerloop_multiple_UAVs_pyramid/Reference_Position ==
  Time_between_quads : Inport
  Clock : Clock
  Gain : Gain
  Gain1 : Gain  Gain=2
  Gain2 : Gain  Gain=3
  Gain3 : Gain  Gain=4
  Gain4 : Gain  Gain=5
  Gain5 : Gain  Gain=6
  Gain6 : Gain  Gain=7
  Gain7 : Gain  Gain=8
  Gain8 : Gain  Gain=9
  Multiport Selector1 : dspindex/Multiport Selector  rowsOrCols=Rows  idxCellArray={1}  idxErrMode=Generate Error
  Multiport Selector10 : dspindex/Multiport Selector  rowsOrCols=Rows  idxCellArray={5}  idxErrMode=Generate Error
  Multiport Selector11 : dspindex/Multiport Selector  rowsOrCols=Rows  idxCellArray={6}  idxErrMode=Generate Error
  Multiport Selector12 : dspindex/Multiport Selector  rowsOrCols=Rows  idxCellArray={6}  idxErrMode=Generate Error
  Multiport Selector13 : dspindex/Multiport Selector  rowsOrCols=Rows  idxCellArray={7}  idxErrMode=Generate Error
  Multiport Selector14 : dspindex/Multiport Selector  rowsOrCols=Rows  idxCellArray={7}  idxErrMode=Generate Error
  Multiport Selector15 : dspindex/Multiport Selector  rowsOrCols=Rows  idxCellArray={8}  idxErrMode=Generate Error
  Multiport Selector16 : dspindex/Multiport Selector  rowsOrCols=Rows  idxCellArray={8}  idxErrMode=Generate Error
  Multiport Selector17 : dspindex/Multiport Selector  rowsOrCols=Rows  idxCellArray={9}  idxErrMode=Generate Error
  Multiport Selector18 : dspindex/Multiport Selector  rowsOrCols=Rows  idxCellArray={9}  idxErrMode=Generate Error
  Multiport Selector2 : dspindex/Multiport Selector  rowsOrCols=Rows  idxCellArray={1}  idxErrMode=Generate Error
  Multiport Selector3 : dspindex/Multiport Selector  rowsOrCols=Rows  idxCellArray={2}  idxErrMode=Generate Error
  Multiport Selector4 : dspindex/Multiport Selector  rowsOrCols=Rows  idxCellArray={2}  idxErrMode=Generate Error
  Multiport Selector5 : dspindex/Multiport Selector  rowsOrCols=Rows  idxCellArray={3}  idxErrMode=Generate Error
  Multiport Selector6 : dspindex/Multiport Selector  rowsOrCols=Rows  idxCellArray={3}  idxErrMode=Generate Error
  Multiport Selector7 : dspindex/Multiport Selector  rowsOrCols=Rows  idxCellArray={4}  idxErrMode=Generate Error
  Multiport Selector8 : dspindex/Multiport Selector  rowsOrCols=Rows  idxCellArray={4}  idxErrMode=Generate Error
  Multiport Selector9 : dspindex/Multiport Selector  rowsOrCols=Rows  idxCellArray={5}  idxErrMode=Generate Error
  Subsystem : Subsystem
  Subsystem1 : Subsystem
  Subsystem2 : Subsystem
  Subsystem3 : Subsystem
  Subsystem4 : Subsystem
  Subsystem5 : Subsystem
  Subsystem6 : Subsystem
  Subsystem7 : Subsystem
  Subsystem8 : Subsystem
  Sum{,1..8} (9 alike) : Sum  Inputs=|+-
  Switch{,1..8} (9 alike) : Switch
  x1 : Constant  Value=Start_POS
  x2 : Constant  Value=End_POS_pyramid
  x3 : Constant  Value=Start_POS
  x4 : Constant  Value=End_POS_pyramid
  x5 : Constant  Value=Start_POS
  x6 : Constant  Value=End_POS_pyramid
  Pos_0 : Outport
  Pos_1 : Outport  Port=2
  Pos_2 : Outport  Port=3
  Pos_3 : Outport  Port=4
  Pos_4 : Outport  Port=5
  Pos_5 : Outport  Port=6
  Pos_6 : Outport  Port=7
  Pos_7 : Outport  Port=8
  Pos_8 : Outport  Port=9
  wires:
  Switch/1 -> Pos_0/1
  Clock/1 -> [SYS_TIME]
  Time_between_quads/1 -> [DeltaT]
  [DeltaT] -> Gain/1
  Gain/1 -> Sum/2
  [SYS_TIME] -> Sum/1
  Sum1/1 -> Subsystem1/1(Time2Maneuver), Switch1/2
  [SYS_TIME] -> Sum1/1
  Gain1/1 -> Sum1/2
  [DeltaT] -> Gain1/1
  Multiport Selector3/1 -> Switch1/1
  Multiport Selector4/1 -> Subsystem1/2(Desired_POS)
  Switch1/1 -> Pos_1/1
  Switch2/1 -> Pos_2/1
  Multiport Selector6/1 -> Subsystem2/2(Desired_POS)
  Multiport Selector5/1 -> Switch2/1
  [DeltaT] -> Gain2/1
  Gain2/1 -> Sum2/2
  [SYS_TIME] -> Sum2/1
  Sum3/1 -> Subsystem3/1(Time2Maneuver), Switch3/2
  [SYS_TIME] -> Sum3/1
  Gain3/1 -> Sum3/2
  [DeltaT] -> Gain3/1
  x1/1 -> Multiport Selector8/1, Multiport Selector6/1, Multiport Selector4/1, Multiport Selector2/1
  x2/1 -> Multiport Selector7/1, Multiport Selector5/1, Multiport Selector3/1, Multiport Selector1/1
  Switch3/1 -> Pos_3/1
  Switch7/1 -> Pos_7/1
  x4/1 -> Multiport Selector15/1, Multiport Selector13/1, Multiport Selector11/1, Multiport Selector9/1
  Multiport Selector15/1 -> Switch7/1
  x3/1 -> Multiport Selector14/1, Multiport Selector16/1, Multiport Selector12/1, Multiport Selector10/1
  [DeltaT] -> Gain7/1
  Gain7/1 -> Sum7/2
  [SYS_TIME] -> Sum7/1
  Sum7/1 -> Subsystem7/1(Time2Maneuver), Switch7/2
  Sum6/1 -> Subsystem6/1(Time2Maneuver), Switch6/2
  [SYS_TIME] -> Sum6/1
  Gain6/1 -> Sum6/2
  [DeltaT] -> Gain6/1
  Multiport Selector13/1 -> Switch6/1
  Switch6/1 -> Pos_6/1
  Switch5/1 -> Pos_5/1
  Multiport Selector11/1 -> Switch5/1
  [DeltaT] -> Gain5/1
  Gain5/1 -> Sum5/2
  [SYS_TIME] -> Sum5/1
  Sum5/1 -> Subsystem5/1(Time2Maneuver), Switch5/2
  Sum4/1 -> Subsystem4/1(Time2Maneuver), Switch4/2
  [SYS_TIME] -> Sum4/1
  Gain4/1 -> Sum4/2
  [DeltaT] -> Gain4/1
  Multiport Selector9/1 -> Switch4/1
  Switch4/1 -> Pos_4/1
  Multiport Selector18/1 -> Switch8/1
  [DeltaT] -> Gain8/1
  Gain8/1 -> Sum8/2
  [SYS_TIME] -> Sum8/1
  Sum8/1 -> Subsystem8/1(Time2Maneuver), Switch8/2
  x5/1 -> Multiport Selector17/1
  x6/1 -> Multiport Selector18/1
  Switch8/1 -> Pos_8/1
  Sum/1 -> Subsystem/1(Time2Maneuver), Switch/2
  Multiport Selector1/1 -> Switch/1
  Multiport Selector2/1 -> Subsystem/2(Desired_POS)
  Subsystem/1(Des_POS) -> Switch/3
  Subsystem1/1(Des_POS) -> Switch1/3
  Sum2/1 -> Subsystem2/1(Time2Maneuver), Switch2/2
  Subsystem2/1(Des_POS) -> Switch2/3
  Multiport Selector8/1 -> Subsystem3/2(Desired_POS)
  Subsystem3/1(Des_POS) -> Switch3/3
  Multiport Selector7/1 -> Switch3/1
  Multiport Selector10/1 -> Subsystem4/2(Desired_POS)
  Multiport Selector12/1 -> Subsystem5/2(Desired_POS)
  Multiport Selector14/1 -> Subsystem6/2(Desired_POS)
  Multiport Selector16/1 -> Subsystem7/2(Desired_POS)
  Multiport Selector17/1 -> Subsystem8/2(Desired_POS)
  Subsystem8/1(Des_POS) -> Switch8/3
  Subsystem4/1(Des_POS) -> Switch4/3
  Subsystem5/1(Des_POS) -> Switch5/3
  Subsystem6/1(Des_POS) -> Switch6/3
  Subsystem7/1(Des_POS) -> Switch7/3

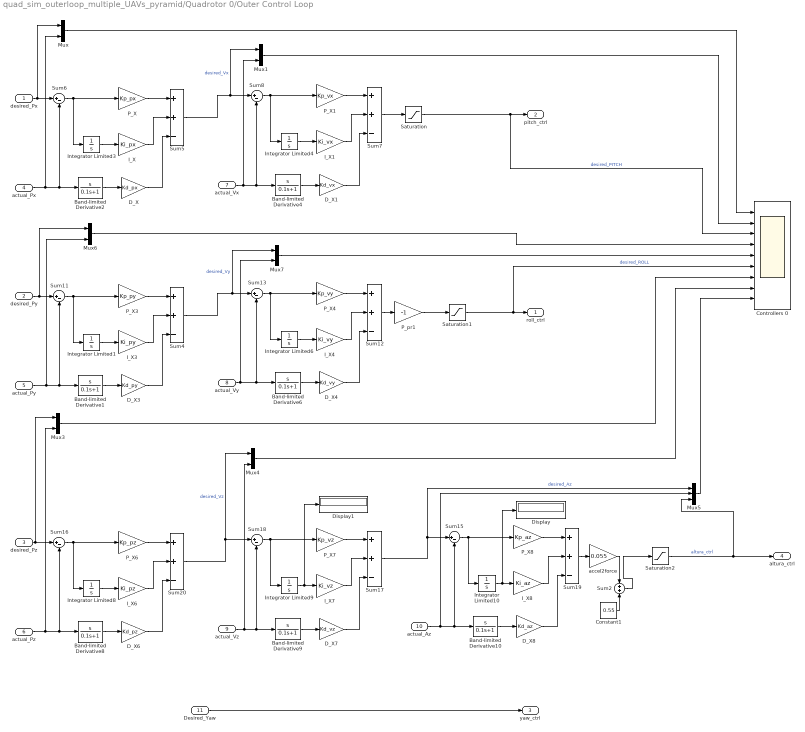
== system quad_sim_outerloop_multiple_UAVs_pyramid/Quadrotor 0/Outer Control Loop ==
  desired_Px : Inport
  desired_Py : Inport  Port=2
  desired_Pz : Inport  Port=3
  actual_Px : Inport  Port=4
  actual_Py : Inport  Port=5
  actual_Pz : Inport  Port=6
  actual_Vx : Inport  Port=7
  actual_Vy : Inport  Port=8
  actual_Vz : Inport  Port=9
  actual_Az : Inport  Port=10
  Desired_Yaw : Inport  Port=11
  Band-limited Derivative{1..2,4,6,8..10} (7 alike) : TransferFcn  Numerator=[1 0]  Denominator=[0.1 1]
  Constant1 : Constant  Value=0.55
  Controllers 0 : Scope  NumInputPorts=9
  D_X : Gain  Gain=Kd_px
  D_X1 : Gain  Gain=Kd_vx
  D_X3 : Gain  Gain=Kd_py
  D_X4 : Gain  Gain=Kd_vy
  D_X6 : Gain  Gain=Kd_pz
  D_X7 : Gain  Gain=Kd_vz
  D_X8 : Gain  Gain=Kd_az
  Display : Display
  Display1 : Display
  I_X : Gain  Gain=Ki_px
  I_X1 : Gain  Gain=Ki_vx
  I_X3 : Gain  Gain=Ki_py
  I_X4 : Gain  Gain=Ki_vy
  I_X6 : Gain  Gain=Ki_pz
  I_X7 : Gain  Gain=Ki_vz
  I_X8 : Gain  Gain=Ki_az
  Integrator Limited{1,3..4,6} (4 alike) : Integrator  LimitOutput=on  UpperSaturationLimit=100  LowerSaturationLimit=-100
  Integrator Limited10 : Integrator  LimitOutput=on  UpperSaturationLimit=1000  LowerSaturationLimit=-1000
  Integrator Limited8 : Integrator  LimitOutput=on  UpperSaturationLimit=1000  LowerSaturationLimit=-1000
  Integrator Limited9 : Integrator  LimitOutput=on  UpperSaturationLimit=1000  LowerSaturationLimit=-1000
  Mux{,1,3..4,6..7} (6 alike) : Mux  Inputs=2
  Mux5 : Mux  Inputs=3
  P_X : Gain  Gain=Kp_px
  P_X1 : Gain  Gain=Kp_vx
  P_X3 : Gain  Gain=Kp_py
  P_X4 : Gain  Gain=Kp_vy
  P_X6 : Gain  Gain=Kp_pz
  P_X7 : Gain  Gain=Kp_vz
  P_X8 : Gain  Gain=Kp_az
  P_pr1 : Gain  Gain=-1
  Saturation : Saturate  UpperLimit=5  LowerLimit=-5
  Saturation1 : Saturate  UpperLimit=5  LowerLimit=-5
  Saturation2 : Saturate  UpperLimit=10  LowerLimit=0
  Sum{6,8,11,13,15..16,18} (7 alike) : Sum  Inputs=|+-
  Sum{4..5,7,12,17,19..20} (7 alike) : Sum  Inputs=++-
  Sum2 : Sum  Inputs=+|+
  accel2force : Gain  Gain=0.055
  roll_ctrl : Outport
  pitch_ctrl : Outport  Port=2
  yaw_ctrl : Outport  Port=3
  altura_ctrl : Outport  Port=4
  wires:
  Desired_Yaw/1 -> yaw_ctrl/1
  Sum6/1 -> Integrator Limited3/1, P_X/1
  Integrator Limited3/1 -> I_X/1
  P_X/1 -> Sum5/1
  D_X/1 -> Sum5/3
  actual_Px/1 -> Mux/2, Band-limited Derivative2/1, Sum6/2
  Band-limited Derivative2/1 -> D_X/1
  I_X/1 -> Sum5/2
  Saturation2/1 -> Mux5/3, altura_ctrl/1  "altura_ctrl"
  Sum8/1 -> P_X1/1, Integrator Limited4/1
  Integrator Limited4/1 -> I_X1/1
  P_X1/1 -> Sum7/1
  D_X1/1 -> Sum7/3
  actual_Vx/1 -> Mux1/2, Sum8/2, Band-limited Derivative4/1
  Band-limited Derivative4/1 -> D_X1/1
  I_X1/1 -> Sum7/2
  Sum5/1 -> Mux1/1, Sum8/1  "desired_Vx"
  Sum7/1 -> Saturation/1
  Sum11/1 -> P_X3/1, Integrator Limited1/1
  Integrator Limited1/1 -> I_X3/1
  P_X3/1 -> Sum4/1
  D_X3/1 -> Sum4/3
  Band-limited Derivative1/1 -> D_X3/1
  I_X3/1 -> Sum4/2
  Sum13/1 -> Integrator Limited6/1, P_X4/1
  Integrator Limited6/1 -> I_X4/1
  P_X4/1 -> Sum12/1
  D_X4/1 -> Sum12/3
  Band-limited Derivative6/1 -> D_X4/1
  I_X4/1 -> Sum12/2
  Sum4/1 -> Sum13/1, Mux7/1  "desired_Vy"
  Sum12/1 -> P_pr1/1
  Sum16/1 -> Integrator Limited8/1, P_X6/1
  Integrator Limited8/1 -> I_X6/1
  P_X6/1 -> Sum20/1
  D_X6/1 -> Sum20/3
  actual_Pz/1 -> Mux3/2, Band-limited Derivative8/1, Sum16/2
  Band-limited Derivative8/1 -> D_X6/1
  I_X6/1 -> Sum20/2
  Sum18/1 -> P_X7/1, Integrator Limited9/1
  Integrator Limited9/1 -> Display1/1, I_X7/1
  P_X7/1 -> Sum17/1
  D_X7/1 -> Sum17/3
  Band-limited Derivative9/1 -> D_X7/1
  I_X7/1 -> Sum17/2
  Sum15/1 -> Integrator Limited10/1, P_X8/1
  Integrator Limited10/1 -> Display/1, I_X8/1
  P_X8/1 -> Sum19/1
  D_X8/1 -> Sum19/3
  Band-limited Derivative10/1 -> D_X8/1
  I_X8/1 -> Sum19/2
  Mux/1 -> Controllers 0/1
  Mux1/1 -> Controllers 0/2
  actual_Vz/1 -> Mux4/2, Sum18/2, Band-limited Derivative9/1
  Sum20/1 -> Mux4/1, Sum18/1  "desired_Vz"
  actual_Az/1 -> Mux5/2, Band-limited Derivative10/1, Sum15/2
  Sum17/1 -> Mux5/1, Sum15/1  "desired_Az"
  Mux3/1 -> Controllers 0/7
  Mux4/1 -> Controllers 0/8
  Sum19/1 -> accel2force/1
  accel2force/1 -> Sum2/1
  Constant1/1 -> Sum2/2
  desired_Py/1 -> Mux6/1, Sum11/1
  actual_Vy/1 -> Band-limited Derivative6/1, Sum13/2, Mux7/2
  Mux6/1 -> Controllers 0/4
  Mux7/1 -> Controllers 0/5
  P_pr1/1 -> Saturation1/1
  Saturation/1 -> Controllers 0/3, pitch_ctrl/1  "desired_PITCH"
  Mux5/1 -> Controllers 0/9
  Saturation1/1 -> Controllers 0/6, roll_ctrl/1  "desired_ROLL"
  desired_Pz/1 -> Mux3/1, Sum16/1
  Sum2/1 -> Saturation2/1
  desired_Px/1 -> Mux/1, Sum6/1
  actual_Py/1 -> Sum11/2, Band-limited Derivative1/1, Mux6/2

== system quad_sim_outerloop_multiple_UAVs_pyramid/Quadrotor 0/Quadrirrotor Communication ==
  roll : Inport
  pitch : Inport  Port=2
  yaw : Inport  Port=3
  throttle : Inport  Port=4
  Blank Message : robotlib/Blank Message  SourceLibraryInfo=This block requires Robotics System Toolbox  messageType=geometry_msgs/Quaternion  SampleTime=inf
      settings: SourceProductBaseCode=RO
  Bus Assignment1 : BusAssignment  DialogController=Simulink.DDGSource_BusAssignment  AssignedSignals=X,Y,Z,W
  Bus Selector1 : BusSelector  OutputSignals=Data
  Data Type Conversion : DataTypeConversion  OutDataTypeStr=double
  Multiport Selector : dspindex/Multiport Selector  rowsOrCols=Rows  idxCellArray={ 1,2,3,4,5,6,7,8,9}  idxErrMode=Generate Error
  Publish2 : robotlib/Publish  SourceLibraryInfo=This block requires Robotics System Toolbox  topicSource=Specify your own  topic=/commands_attitude_0  messageType=geometry_msgs/Quaternion  messageQueueLength=105
      settings: SourceProductBaseCode=RO
  Subscribe : robotlib/Subscribe  SourceLibraryInfo=This block requires Robotics System Toolbox  topicSource=Specify your own  topic=/quadrotor_states_0  messageType=std_msgs/Float32MultiArray  sampleTime=-1  messageQueueLength=51
      settings: SourceProductBaseCode=RO
  Terminator : Terminator
  quad_pos_x : Outport
  quad_pos_y : Outport  Port=2
  quad_pos_z : Outport  Port=3
  quad_vel_x : Outport  Port=4
  quad_vel_y : Outport  Port=5
  quad_vel_z : Outport  Port=6
  quad_acc_x : Outport  Port=7
  quad_acc_y : Outport  Port=8
  quad_acc_z : Outport  Port=9
  wires:
  Blank Message/1 -> Bus Assignment1/1
  Subscribe/1 -> Terminator/1
  Subscribe/2 -> Bus Selector1/1
  Bus Assignment1/1 -> Publish2/1
  Multiport Selector/1 -> quad_pos_x/1
  Multiport Selector/2 -> quad_pos_y/1
  Multiport Selector/3 -> quad_pos_z/1
  Multiport Selector/4 -> quad_vel_x/1
  Multiport Selector/5 -> quad_vel_y/1
  Multiport Selector/6 -> quad_vel_z/1
  Multiport Selector/7 -> quad_acc_x/1
  Multiport Selector/8 -> quad_acc_y/1
  Multiport Selector/9 -> quad_acc_z/1
  Data Type Conversion/1 -> Multiport Selector/1
  Bus Selector1/1 -> Data Type Conversion/1  "<Data>"
  throttle/1 -> Bus Assignment1/5
  yaw/1 -> Bus Assignment1/4
  pitch/1 -> Bus Assignment1/3
  roll/1 -> Bus Assignment1/2

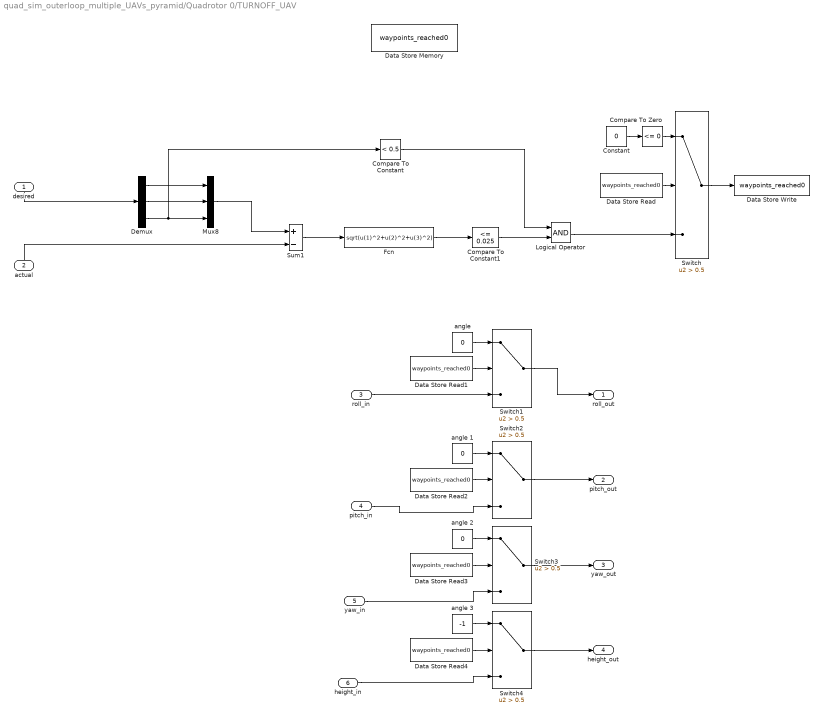
== system quad_sim_outerloop_multiple_UAVs_pyramid/Quadrotor 0/TURNOFF_UAV ==
  desired : Inport
  actual : Inport  Port=2
  roll_in : Inport  Port=3
  pitch_in : Inport  Port=4
  yaw_in : Inport  Port=5
  height_in : Inport  Port=6
  Compare To Constant : simulink/Logic and Bit Operations/Compare To Constant  relop=<  const=0.5  OutDataTypeStr=boolean
  Compare To Constant1 : simulink/Logic and Bit Operations/Compare To Constant  relop=<=  const=0.025  OutDataTypeStr=boolean
  Compare To Zero : simulink/Logic and Bit Operations/Compare To Zero  relop=<=  OutDataTypeStr=boolean
  Constant : Constant  Value=0
  Data Store Memory : DataStoreMemory  DataStoreName=waypoints_reached0  ShowAdditionalParam=off  OutDataTypeStr=boolean
  Data Store Read{,1..4} (5 alike) : DataStoreRead  DataStoreName=waypoints_reached0
  Data Store Write : DataStoreWrite  DataStoreName=waypoints_reached0
  Demux : Demux  Outputs=3
  Fcn : Fcn  Expr=sqrt(u(1)^2+u(2)^2+u(3)^2)
  Logical Operator : Logic  AllPortsSameDT=off  OutDataTypeStr=boolean
  Mux8 : Mux  Inputs=3
  Sum1 : Sum  Inputs=+-
  Switch{,1..4} (5 alike) : Switch  Criteria=u2 > Threshold  Threshold=0.5
  "angle " : Constant  Value=0
  angle 1 : Constant  Value=0
  angle 2 : Constant  Value=0
  angle 3 : Constant  Value=-1
  roll_out : Outport
  pitch_out : Outport  Port=2
  yaw_out : Outport  Port=3
  height_out : Outport  Port=4
  wires:
  roll_in/1 -> Switch1/3
  pitch_in/1 -> Switch2/3
  angle 2/1 -> Switch3/1
  yaw_in/1 -> Switch3/3
  "angle "/1 -> Switch1/1
  angle 1/1 -> Switch2/1
  height_in/1 -> Switch4/3
  Switch2/1 -> pitch_out/1
  Switch1/1 -> roll_out/1
  Demux/2 -> Mux8/2
  Demux/3 -> Mux8/3, Compare To Constant/1
  Logical Operator/1 -> Switch/3
  Compare To Constant/1 -> Logical Operator/1
  Compare To Constant1/1 -> Logical Operator/2
  Sum1/1 -> Fcn/1
  Fcn/1 -> Compare To Constant1/1
  Mux8/1 -> Sum1/1
  Compare To Zero/1 -> Switch/1
  Data Store Read2/1 -> Switch2/2
  Data Store Read4/1 -> Switch4/2
  Data Store Read1/1 -> Switch1/2
  Switch/1 -> Data Store Write/1
  Data Store Read3/1 -> Switch3/2
  angle 3/1 -> Switch4/1
  Switch3/1 -> yaw_out/1
  Switch4/1 -> height_out/1
  Data Store Read/1 -> Switch/2
  Constant/1 -> Compare To Zero/1
  Demux/1 -> Mux8/1
  desired/1 -> Demux/1
  actual/1 -> Sum1/2
